simulink model "p53_mdm2_simulation_simulink"  (R2024a)
settings: Solver=ode15s  StartTime=0.0  StopTime=60  MaxStep=0.1  RelTol=1e-8  AbsTol=1e-8
model workspace (MAT data in the model file):
  x = Simulink.Parameter
  x.Complexity = 'real'
  x.Dimensions = [0 0]
  x.DataType = 'auto'
values from neighbouring files (symbols this model uses):
  dx = positions(i, 5)    [PSO_5_params.m]    (also in PSO_6_params.m; p53_mdm2_simulation.m = 1; params.m = 1; plot_theoretical_pso_params.m = gBest(5))
  dy = positions(i, 6)    [PSO_6_params.m]    (also in p53_mdm2_simulation.m = 1; params.m = 1; plot_theoretical_pso_params.m = gBest(6))
  K1 = 0.1    [p53_mdm2_simulation.m]    (also in params.m)
  k1 = positions(i, 1)    [PSO.m]    (also in PSO_3_params.m; PSO_4_params.m; PSO_5_params.m; PSO_6_params.m)
  K2 = 1    [p53_mdm2_simulation.m]    (also in params.m)
  k2 = positions(i, 2)    [PSO.m]    (also in PSO_3_params.m; PSO_4_params.m; PSO_5_params.m; PSO_6_params.m)
  ks = 2    [p53_mdm2_simulation.m]    (also in params.m)
  n = positions(i,4)    [PSO_4_params.m]    (also in PSO_5_params.m = positions(i, 4); PSO_6_params.m = positions(i, 4); p53_mdm2_simulation.m = 2; params.m = 2)
  tau = positions(i, 3)    [PSO.m]    (also in PSO_3_params.m; PSO_4_params.m; PSO_5_params.m; PSO_6_params.m)
settings Model: Creator=shirley  LastModifiedBy=shirley

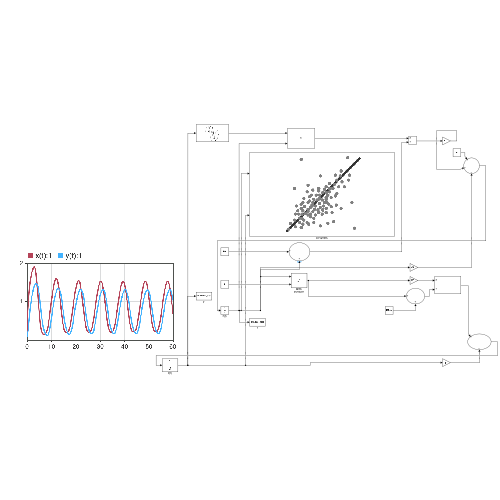
[thumbnail: Simulink's stored preview of the top-level diagram]
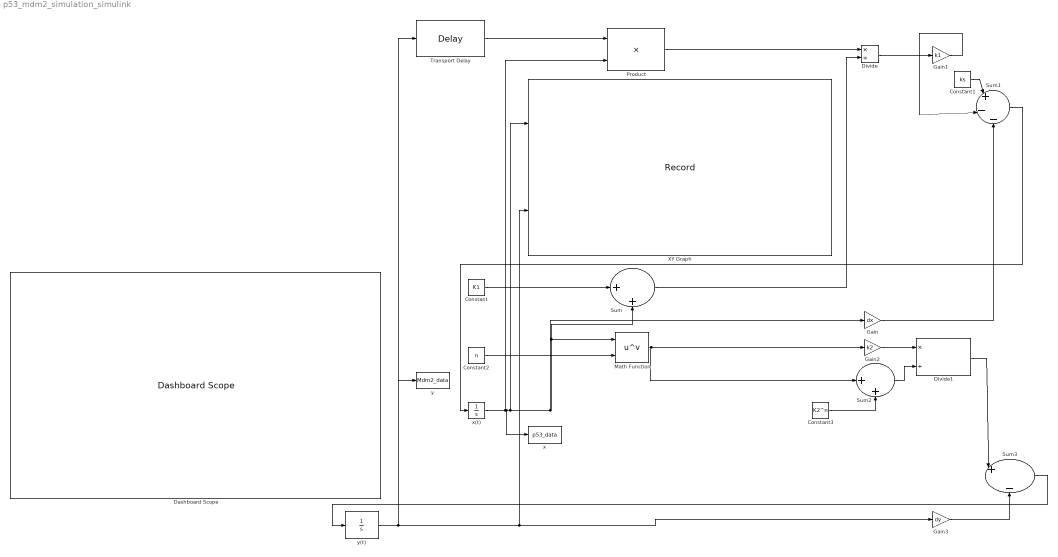
== system p53_mdm2_simulation_simulink ==
  Constant : Constant  Value=K1
  Constant1 : Constant  Value=ks
  Constant2 : Constant  Value=n
  Constant3 : Constant  Value=K2^n
  Dashboard Scope : DashboardScope
  Divide : Product  Inputs=*/
  Divide1 : Product  Inputs=*/
  Gain : Gain  Gain=dx
  Gain1 : Gain  Gain=k1
  Gain2 : Gain  Gain=k2
  Gain3 : Gain  Gain=dy
  Math Function : Math  Operator=pow
  Product : Product
  Sum : Sum  Inputs=|++
  Sum1 : Sum  Inputs=|+|-|-
  Sum2 : Sum  Inputs=|++
  Sum3 : Sum  Inputs=|+|-
  Transport Delay : TransportDelay  DelayTime=tau
  XY Graph : Record  FileSettingsInternal="{\"entries\":[{\"content\":{\"excelSettings\":{\"content\":{},\"type\":\"Streamout.ExcelSettings\"}},\"type\":\"Streamout.FileSettingStorage\",\"uuid\":\"\"}],\"packageUris\":[\"http:\\/\\/schema.mathworks.com\\/mf0\\/streamout_blocks\\/R2020a\"],\"version\":\"1.0\"}"  Layout=[1 1]  SignalsInternal="{\"entries\":[{\"content\":{\"signals\":[{\"content\":{\"blockPath\":[],\"dimensions\":[1],\"domain\":\"\",\"lineColor\":\"#a2142f\",\"plots\":[ 1 ],\"port\":1,\"sid\":[\"\"],\"signalID\":1,\"signalName\":\"x(t)\"},\"type\":\"RecordBlkView.Signal\",\"uuid\":\"\"},{\"content\":{\"blockPath\":[],\"dimensions\":[1],\"domain\":\"\",\"lineColor\":\"#139fff\",\"plots\":[ 1 ],\"port\":2,\"sid\":[\"\"],\"signalID\":2,\"signalName\":\"y(t)\"},\"type\":\"RecordBlkView.Signal\",\"uuid\":\"\"}]},\"type\":\"RecordBlkView.InputSignals\",\"uuid\":\"\"}],\"packageUris\":[\"http:\\/\\/schema.mathworks.com\\/mf0\\/streamout_blocks\\/R2020a\"],\"version\":\"1.0\"}"  VisualizationBindings="{\"xyplotplugin\":{\"info\":[{\"series\":[{\"bindingParametersList\":[{\"parameter\":\"X-Axis\",\"signalID\":1,\"signalName\":\"x(t)\"},{\"parameter\":\"Y-Axis\",\"signalID\":2,\"signalName\":\"y(t)\"}],\"seriesID\":0}],\"subplotID\":1}]}}"  CompatibilityTag=XY
  x : ToWorkspace  VariableName=p53_data  SampleTime=-1
  x(t) : Integrator  InitialCondition=0.2  ContinuousStateAttributes="\"x\""
  y : ToWorkspace  VariableName=Mdm2_data  SampleTime=-1
  y(t) : Integrator  InitialCondition=0.1  ContinuousStateAttributes="\"y\""
  wires:
  Sum1/1 -> x(t)/1
  Divide1/1 -> Sum3/1
  Gain1/1 -> Sum1/2
  Constant1/1 -> Sum1/1
  Sum2/1 -> Divide1/2
  Gain2/1 -> Divide1/1
  Gain/1 -> Sum1/3
  Math Function/1 -> Sum2/1, Gain2/1
  Sum3/1 -> y(t)/1
  x(t)/1 -> Math Function/1, Sum/2, Gain/1, XY Graph/1, x/1, Product/2
  Constant3/1 -> Sum2/2
  Sum/1 -> Divide/2
  Product/1 -> Divide/1
  Transport Delay/1 -> Product/1
  Divide/1 -> Gain1/1
  y(t)/1 -> Gain3/1, XY Graph/2, Transport Delay/1, y/1
  Gain3/1 -> Sum3/2
  Constant2/1 -> Math Function/2
  Constant/1 -> Sum/1
